simulink model "Adaptive_Controller_withoutDisturbance"  (R2021a)
settings: Solver=VariableStepAuto  StartTime=0.0  StopTime=1200  RelTol=1e-3
settings Model: SimulationMode=rapid-accelerator  Creator=sahil  LastModifiedBy=sahil

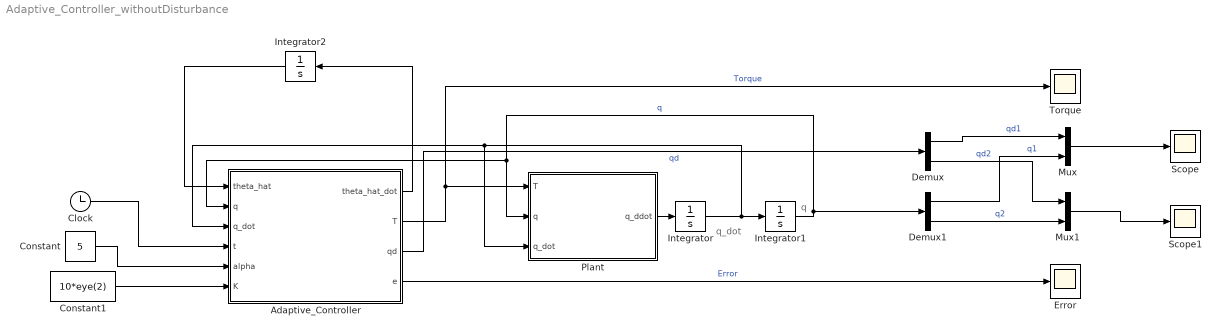
== system Adaptive_Controller_withoutDisturbance ==
  note: q
  note: q_dot
  Adaptive_Controller : MATLAB Function  TreatAsAtomicUnit=on
  Clock : Clock
  Constant : Constant  Value=5
  Constant1 : Constant  Value=10*eye(2)
  Demux : Demux  Outputs=2
  Demux1 : Demux  Outputs=2
  Error : Scope
  Integrator : Integrator  InitialCondition=[0; 0]
  Integrator1 : Integrator  InitialCondition=[0; 0]
  Integrator2 : Integrator  InitialCondition=[0;0;0;0]
  Mux : Mux  Inputs=2
  Mux1 : Mux  Inputs=2
  Plant : MATLAB Function  TreatAsAtomicUnit=on
  Scope : Scope
  Scope1 : Scope
  Torque : Scope
  wires:
  Integrator1/1 -> Demux1/1, Plant/2(q), Adaptive_Controller/2(q)  "q"
  Clock/1 -> Adaptive_Controller/4(t)
  Constant/1 -> Adaptive_Controller/5(alpha)
  Plant/1(q_ddot) -> Integrator/1
  Integrator/1 -> Plant/3(q_dot), Adaptive_Controller/3(q_dot), Integrator1/1
  Adaptive_Controller/4(e) -> Error/1  "Error"
  Demux1/2 -> Mux1/2  "q2"
  Adaptive_Controller/2(T) -> Torque/1, Plant/1(T)  "Torque"
  Demux/2 -> Mux1/1  "qd2"
  Mux/1 -> Scope/1
  Demux1/1 -> Mux/2  "q1"
  Adaptive_Controller/3(qd) -> Demux/1  "qd"
  Demux/1 -> Mux/1  "qd1"
  Constant1/1 -> Adaptive_Controller/6(K)
  Mux1/1 -> Scope1/1
  Adaptive_Controller/1(theta_hat_dot) -> Integrator2/1
  Integrator2/1 -> Adaptive_Controller/1(theta_hat)

== matlab function Adaptive_Controller_withoutDisturbance/Adaptive_Controller ==
  data: theta_hat input; theta_hat_dot output; q input; q_dot input; t input; T output; qd output; e output; alpha input; K input
function [theta_hat_dot, T, qd, e] = fcn(theta_hat, q, q_dot, t, alpha, K)
%Defining given parameters
p1 = 3.473;
p2 = 0.196;
p3 = 0.242;
fd1 = 5.3;
fd2 = 1.1;

%Defining Robot Dynamic Model
M = [(p1 + 2*p3*cos(q(2))) (p2 + p3*cos(q(2))); (p2 + p3*cos(q(2))) p2];
Vm = [(-p3*sin(q(2))*q_dot(2)) (-p3*sin(q(2))*(q_dot(1)+q_dot(2))); (p3*sin(q(2))*q_dot(1)) 0];
Fd = [fd1 0; 0 fd2];

%Control Gains
% K = 5*eye(2);

%Defining Desired trajectories
qd = [cos(t); cos(2*t)];
qd_dot = [-sin(t); -2*sin(2*t)];
qd_ddot = [-cos(t); -4*cos(2*t)];

%Defining Errors
e = qd - q;
e_dot = qd_dot - q_dot;
r = e_dot + (alpha*e);

%Adaptive Controller
Gamma = eye(4);
Y = [qd_ddot,qd_dot+alpha*e,q_dot,alpha*e_dot]
theta_hat_dot = (inv(Gamma))*(Y')*r;
T = (Y*theta_hat) + e+ (K*r);

== matlab function Adaptive_Controller_withoutDisturbance/Plant ==
  data: T input; q_ddot output; q input; q_dot input
function q_ddot = fcn(T, q, q_dot)

%Defining given parameters
p1 = 3.473;
p2 = 0.196;
p3 = 0.242;
fd1 = 5.3;
fd2 = 1.1;

%Defining Robot Dynamic Model
M = [(p1 + 2*p3*cos(q(2))) (p2 + p3*cos(q(2))); (p2 + p3*cos(q(2))) p2];
Vm = [(-p3*sin(q(2))*q_dot(2)) (-p3*sin(q(2))*(q_dot(1)+q_dot(2))); (p3*sin(q(2))*q_dot(1)) 0];
Fd = [fd1 0; 0 fd2];

%Robot Dynamics
q_ddot = inv(M)*(T - (Vm*q_dot) - (Fd*q_dot));
